simulink model "gm_UZ_EnDat_be4_segregation"  (R2023b)
settings: Solver=FixedStepAuto  StartTime=0  StopTime=0.000505  RelTol=1e-3
model workspace (MAT data in the model file):
  Select = 0
libraries: hdlsllib x74, simulink x21, hdlmdlgenlib x4, simulink_extras x1
(part 4 of 5)

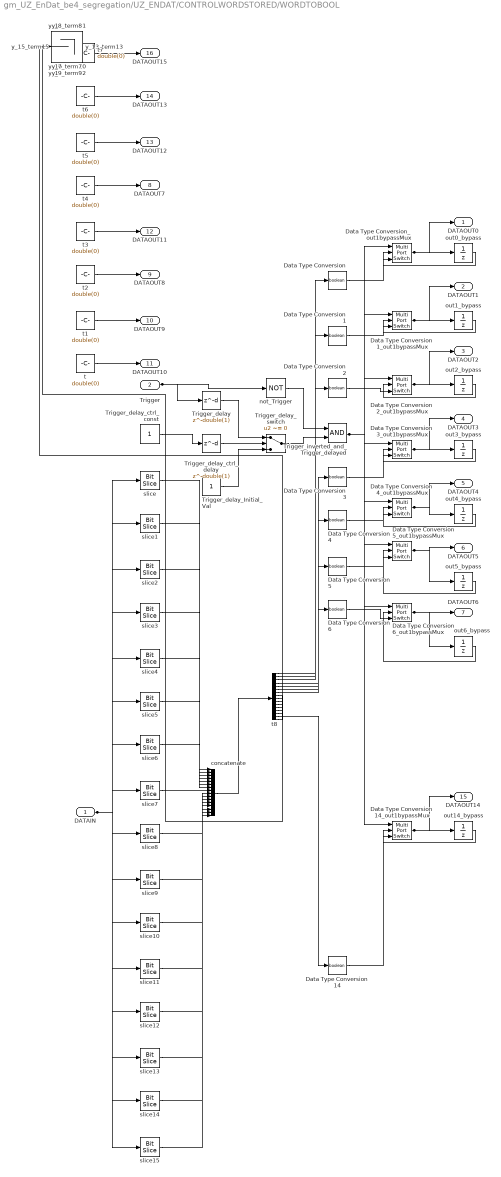
== system gm_UZ_EnDat_be4_segregation/UZ_ENDAT/CONTROLWORDSTORED/WORDTOBOOL ==
  DATAIN : Inport  OutDataTypeStr=uint16  PortDimensions=1  SampleTime=1e-08
  Trigger : Inport  Port=2  OutDataTypeStr=boolean  SampleTime=1e-08
  Data Type Conversion{,1..6,14} (8 alike) : DataTypeConversion  OutDataTypeStr=boolean  SampleTime=1e-08  SaturateOnIntegerOverflow=off  RndMeth=Floor
  Data Type Conversion14_out1bypassMux : MultiPortSwitch  DataPortOrder=Zero-based contiguous  Inputs=2  zeroidx=on  SampleTime=1e-08  SaturateOnIntegerOverflow=off  InputSameDT=off
  Data Type Conversion1_out1bypassMux : MultiPortSwitch  DataPortOrder=Zero-based contiguous  Inputs=2  zeroidx=on  SampleTime=1e-08  SaturateOnIntegerOverflow=off  InputSameDT=off
  Data Type Conversion2_out1bypassMux : MultiPortSwitch  DataPortOrder=Zero-based contiguous  Inputs=2  zeroidx=on  SampleTime=1e-08  SaturateOnIntegerOverflow=off  InputSameDT=off
  Data Type Conversion3_out1bypassMux : MultiPortSwitch  DataPortOrder=Zero-based contiguous  Inputs=2  zeroidx=on  SampleTime=1e-08  SaturateOnIntegerOverflow=off  InputSameDT=off
  Data Type Conversion4_out1bypassMux : MultiPortSwitch  DataPortOrder=Zero-based contiguous  Inputs=2  zeroidx=on  SampleTime=1e-08  SaturateOnIntegerOverflow=off  InputSameDT=off
  Data Type Conversion5_out1bypassMux : MultiPortSwitch  DataPortOrder=Zero-based contiguous  Inputs=2  zeroidx=on  SampleTime=1e-08  SaturateOnIntegerOverflow=off  InputSameDT=off
  Data Type Conversion6_out1bypassMux : MultiPortSwitch  DataPortOrder=Zero-based contiguous  Inputs=2  zeroidx=on  SampleTime=1e-08  SaturateOnIntegerOverflow=off  InputSameDT=off
  Data Type Conversion_out1bypassMux : MultiPortSwitch  DataPortOrder=Zero-based contiguous  Inputs=2  zeroidx=on  SampleTime=1e-08  SaturateOnIntegerOverflow=off  InputSameDT=off
  Trigger_delay : Delay  DelayLength=double(1)  InitialCondition=0
  Trigger_delay_Initial_Val : Constant  OutDataTypeStr=boolean  SampleTime=1e-08
  Trigger_delay_ctrl_const : Constant  OutDataTypeStr=boolean  SampleTime=1e-08
  Trigger_delay_ctrl_delay : Delay  DelayLength=double(1)  InitialCondition=0
  Trigger_delay_switch : Switch  Criteria=u2 ~= 0  Threshold=double(0)  OutDataTypeStr=boolean  SampleTime=1e-08  SaturateOnIntegerOverflow=off  InputSameDT=off
  Trigger_inverted_and_Trigger_delayed : Logic  AllPortsSameDT=off  OutDataTypeStr=boolean  SampleTime=1e-08
  concatenate : Concatenate  NumInputs=16  Mode=Multidimensional array  ConcatenateDimension=2
  not_Trigger : Logic  Operator=NOT  Inputs=1  AllPortsSameDT=off  OutDataTypeStr=boolean  SampleTime=1e-08
  out0_bypass : UnitDelay  SampleTime=1e-08
  out14_bypass : UnitDelay  SampleTime=1e-08
  out1_bypass : UnitDelay  SampleTime=1e-08
  out2_bypass : UnitDelay  SampleTime=1e-08
  out3_bypass : UnitDelay  SampleTime=1e-08
  out4_bypass : UnitDelay  SampleTime=1e-08
  out5_bypass : UnitDelay  SampleTime=1e-08
  out6_bypass : UnitDelay  SampleTime=1e-08
  slice : hdlsllib/Logic and Bit Operations/Bit Slice  lidx=double(0)  ridx=double(0)
  slice1 : hdlsllib/Logic and Bit Operations/Bit Slice  lidx=double(1)  ridx=double(1)
  slice10 : hdlsllib/Logic and Bit Operations/Bit Slice  lidx=double(10)  ridx=double(10)
  slice11 : hdlsllib/Logic and Bit Operations/Bit Slice  lidx=double(11)  ridx=double(11)
  slice12 : hdlsllib/Logic and Bit Operations/Bit Slice  lidx=double(12)  ridx=double(12)
  slice13 : hdlsllib/Logic and Bit Operations/Bit Slice  lidx=double(13)  ridx=double(13)
  slice14 : hdlsllib/Logic and Bit Operations/Bit Slice  lidx=double(14)  ridx=double(14)
  slice15 : hdlsllib/Logic and Bit Operations/Bit Slice  lidx=double(15)  ridx=double(15)
  slice2 : hdlsllib/Logic and Bit Operations/Bit Slice  lidx=double(2)  ridx=double(2)
  slice3 : hdlsllib/Logic and Bit Operations/Bit Slice  lidx=double(3)  ridx=double(3)
  slice4 : hdlsllib/Logic and Bit Operations/Bit Slice  lidx=double(4)  ridx=double(4)
  slice5 : hdlsllib/Logic and Bit Operations/Bit Slice  lidx=double(5)  ridx=double(5)
  slice6 : hdlsllib/Logic and Bit Operations/Bit Slice  lidx=double(6)  ridx=double(6)
  slice7 : hdlsllib/Logic and Bit Operations/Bit Slice  lidx=double(7)  ridx=double(7)
  slice8 : hdlsllib/Logic and Bit Operations/Bit Slice  lidx=double(8)  ridx=double(8)
  slice9 : hdlsllib/Logic and Bit Operations/Bit Slice  lidx=double(9)  ridx=double(9)
  t{,1..7} (8 alike) : Constant  Value=double(0)  OutDataTypeStr=boolean  SampleTime=1e-08
  t8 : Demux  Outputs=16
  y_10_term10 : Terminator
  y_11_term11 : Terminator
  y_12_term12 : Terminator
  y_13_term13 : Terminator
  y_15_term15 : Terminator
  y_7_term7 : Terminator
  y_8_term8 : Terminator
  y_9_term9 : Terminator
  DATAOUT0 : Outport  SampleTime=1e-08  InitialOutput=0
  DATAOUT1 : Outport  Port=2  SampleTime=1e-08  InitialOutput=0
  DATAOUT2 : Outport  Port=3  SampleTime=1e-08  InitialOutput=0
  DATAOUT3 : Outport  Port=4  SampleTime=1e-08  InitialOutput=0
  DATAOUT4 : Outport  Port=5  SampleTime=1e-08  InitialOutput=0
  DATAOUT5 : Outport  Port=6  SampleTime=1e-08  InitialOutput=0
  DATAOUT6 : Outport  Port=7  SampleTime=1e-08  InitialOutput=0
  DATAOUT7 : Outport  Port=8  SampleTime=1e-08  InitialOutput=0
  DATAOUT8 : Outport  Port=9  SampleTime=1e-08  InitialOutput=0
  DATAOUT9 : Outport  Port=10  SampleTime=1e-08  InitialOutput=0
  DATAOUT10 : Outport  Port=11  SampleTime=1e-08  InitialOutput=0
  DATAOUT11 : Outport  Port=12  SampleTime=1e-08  InitialOutput=0
  DATAOUT12 : Outport  Port=13  SampleTime=1e-08  InitialOutput=0
  DATAOUT13 : Outport  Port=14  SampleTime=1e-08  InitialOutput=0
  DATAOUT14 : Outport  Port=15  SampleTime=1e-08  InitialOutput=0
  DATAOUT15 : Outport  Port=16  SampleTime=1e-08  InitialOutput=0
  wires:
  Trigger/1 -> not_Trigger/1, Trigger_delay/1
  DATAIN/1 -> slice15/1, slice14/1, slice13/1, slice12/1, slice11/1, slice10/1, slice9/1, slice8/1, slice7/1, slice6/1, slice5/1, slice4/1, slice3/1, slice2/1, slice1/1, slice/1
  Data Type Conversion_out1bypassMux/1 -> DATAOUT0/1, out0_bypass/1
  Data Type Conversion1_out1bypassMux/1 -> DATAOUT1/1, out1_bypass/1
  Data Type Conversion2_out1bypassMux/1 -> DATAOUT2/1, out2_bypass/1
  Data Type Conversion3_out1bypassMux/1 -> DATAOUT3/1, out3_bypass/1
  Data Type Conversion4_out1bypassMux/1 -> DATAOUT4/1, out4_bypass/1
  Data Type Conversion5_out1bypassMux/1 -> DATAOUT5/1, out5_bypass/1
  Data Type Conversion6_out1bypassMux/1 -> DATAOUT6/1, out6_bypass/1
  t4/1 -> DATAOUT7/1
  t2/1 -> DATAOUT8/1
  t1/1 -> DATAOUT9/1
  t/1 -> DATAOUT10/1
  t3/1 -> DATAOUT11/1
  t5/1 -> DATAOUT12/1
  t6/1 -> DATAOUT13/1
  Data Type Conversion14_out1bypassMux/1 -> DATAOUT14/1, out14_bypass/1
  t7/1 -> DATAOUT15/1
  Trigger_delay_switch/1 -> Trigger_inverted_and_Trigger_delayed/2
  not_Trigger/1 -> Trigger_inverted_and_Trigger_delayed/1
  Trigger_inverted_and_Trigger_delayed/1 -> Data Type Conversion_out1bypassMux/1, Data Type Conversion1_out1bypassMux/1, Data Type Conversion2_out1bypassMux/1, Data Type Conversion3_out1bypassMux/1, Data Type Conversion4_out1bypassMux/1, Data Type Conversion5_out1bypassMux/1, Data Type Conversion6_out1bypassMux/1, Data Type Conversion14_out1bypassMux/1
  Trigger_delay/1 -> Trigger_delay_switch/1
  Trigger_delay_Initial_Val/1 -> Trigger_delay_switch/3
  Trigger_delay_ctrl_delay/1 -> Trigger_delay_switch/2
  concatenate/1 -> t8/1
  t8/1 -> Data Type Conversion/1
  t8/2 -> Data Type Conversion1/1
  t8/3 -> Data Type Conversion2/1
  t8/4 -> Data Type Conversion3/1
  t8/5 -> Data Type Conversion4/1
  t8/6 -> Data Type Conversion5/1
  t8/7 -> Data Type Conversion6/1
  t8/8 -> y_7_term7/1
  t8/9 -> y_8_term8/1
  t8/10 -> y_9_term9/1
  t8/11 -> y_10_term10/1
  t8/12 -> y_11_term11/1
  t8/13 -> y_12_term12/1
  t8/14 -> y_13_term13/1
  t8/15 -> Data Type Conversion14/1
  t8/16 -> y_15_term15/1
  slice/1 -> concatenate/1
  slice1/1 -> concatenate/2
  slice2/1 -> concatenate/3
  slice3/1 -> concatenate/4
  slice4/1 -> concatenate/5
  slice5/1 -> concatenate/6
  slice6/1 -> concatenate/7
  slice7/1 -> concatenate/8
  slice8/1 -> concatenate/9
  slice9/1 -> concatenate/10
  slice10/1 -> concatenate/11
  slice11/1 -> concatenate/12
  slice12/1 -> concatenate/13
  slice13/1 -> concatenate/14
  slice14/1 -> concatenate/15
  slice15/1 -> concatenate/16
  out14_bypass/1 -> Data Type Conversion14_out1bypassMux/2
  Data Type Conversion14/1 -> Data Type Conversion14_out1bypassMux/3
  out0_bypass/1 -> Data Type Conversion_out1bypassMux/2
  Data Type Conversion/1 -> Data Type Conversion_out1bypassMux/3
  out1_bypass/1 -> Data Type Conversion1_out1bypassMux/2
  Data Type Conversion1/1 -> Data Type Conversion1_out1bypassMux/3
  out2_bypass/1 -> Data Type Conversion2_out1bypassMux/2
  Data Type Conversion2/1 -> Data Type Conversion2_out1bypassMux/3
  out3_bypass/1 -> Data Type Conversion3_out1bypassMux/2
  Data Type Conversion3/1 -> Data Type Conversion3_out1bypassMux/3
  out4_bypass/1 -> Data Type Conversion4_out1bypassMux/2
  Data Type Conversion4/1 -> Data Type Conversion4_out1bypassMux/3
  out5_bypass/1 -> Data Type Conversion5_out1bypassMux/2
  Data Type Conversion5/1 -> Data Type Conversion5_out1bypassMux/3
  out6_bypass/1 -> Data Type Conversion6_out1bypassMux/2
  Data Type Conversion6/1 -> Data Type Conversion6_out1bypassMux/3
  Trigger_delay_ctrl_const/1 -> Trigger_delay_ctrl_delay/1

== system gm_UZ_EnDat_be4_segregation/UZ_ENDAT/CRC_Check/FF0 ==
  S : Inport  OutDataTypeStr=boolean  PortDimensions=1  SampleTime=1e-08
  CLK : Inport  Port=2  OutDataTypeStr=boolean  PortDimensions=1  SampleTime=1e-08
  DATA : Inport  Port=3  OutDataTypeStr=boolean  PortDimensions=1  SampleTime=1e-08
  R : Inport  Port=4  OutDataTypeStr=boolean  PortDimensions=1  SampleTime=1e-08
  Delay{,1..5} (6 alike) : Delay  DelayLength=double(1)  InitialCondition=0  SampleTime=1e-08
  Logical Operator{,1..5} (6 alike) : Logic  Operator=NAND  Inputs=3  AllPortsSameDT=off  OutDataTypeStr=boolean  SampleTime=1e-08
  Q : Outport  SampleTime=1e-08
  NQ : Outport  Port=2  SampleTime=1e-08
  wires:
  S/1 -> Logical Operator/1, Logical Operator4/1
  CLK/1 -> Logical Operator1/2, Logical Operator2/2
  R/1 -> Logical Operator3/3, Logical Operator1/3, Logical Operator5/3
  Delay1/1 -> Logical Operator/3, Logical Operator2/1, Logical Operator4/2
  Delay2/1 -> Logical Operator3/1, Logical Operator5/2
  Delay4/1 -> Q/1, Logical Operator5/1
  Delay5/1 -> NQ/1, Logical Operator4/3
  Delay3/1 -> Logical Operator/2, Logical Operator2/3
  Logical Operator2/1 -> Delay2/1
  Logical Operator3/1 -> Delay3/1
  DATA/1 -> Logical Operator3/2
  Logical Operator/1 -> Delay/1
  Logical Operator1/1 -> Delay1/1
  Delay/1 -> Logical Operator1/1
  Logical Operator5/1 -> Delay5/1
  Logical Operator4/1 -> Delay4/1

== system gm_UZ_EnDat_be4_segregation/UZ_ENDAT/CRC_Check/FF1 ==
  S : Inport  OutDataTypeStr=boolean  PortDimensions=1  SampleTime=1e-08
  CLK : Inport  Port=2  OutDataTypeStr=boolean  PortDimensions=1  SampleTime=1e-08
  DATA : Inport  Port=3  OutDataTypeStr=boolean  PortDimensions=1  SampleTime=1e-08
  R : Inport  Port=4  OutDataTypeStr=boolean  PortDimensions=1  SampleTime=1e-08
  Delay{,1..5} (6 alike) : Delay  DelayLength=double(1)  InitialCondition=0  SampleTime=1e-08
  Logical Operator{,1..5} (6 alike) : Logic  Operator=NAND  Inputs=3  AllPortsSameDT=off  OutDataTypeStr=boolean  SampleTime=1e-08
  Q : Outport  SampleTime=1e-08
  NQ : Outport  Port=2  SampleTime=1e-08
  wires:
  Logical Operator4/1 -> Delay4/1
  Logical Operator5/1 -> Delay5/1
  Delay/1 -> Logical Operator1/1
  Logical Operator1/1 -> Delay1/1
  Logical Operator/1 -> Delay/1
  DATA/1 -> Logical Operator3/2
  Logical Operator3/1 -> Delay3/1
  Logical Operator2/1 -> Delay2/1
  Delay3/1 -> Logical Operator2/3, Logical Operator/2
  Delay5/1 -> Logical Operator4/3, NQ/1
  Delay4/1 -> Logical Operator5/1, Q/1
  Delay2/1 -> Logical Operator5/2, Logical Operator3/1
  Delay1/1 -> Logical Operator4/2, Logical Operator2/1, Logical Operator/3
  R/1 -> Logical Operator5/3, Logical Operator1/3, Logical Operator3/3
  CLK/1 -> Logical Operator2/2, Logical Operator1/2
  S/1 -> Logical Operator4/1, Logical Operator/1

== system gm_UZ_EnDat_be4_segregation/UZ_ENDAT/CRC_Check/FF2 ==
  S : Inport  OutDataTypeStr=boolean  PortDimensions=1  SampleTime=1e-08
  CLK : Inport  Port=2  OutDataTypeStr=boolean  PortDimensions=1  SampleTime=1e-08
  DATA : Inport  Port=3  OutDataTypeStr=boolean  PortDimensions=1  SampleTime=1e-08
  R : Inport  Port=4  OutDataTypeStr=boolean  PortDimensions=1  SampleTime=1e-08
  Delay{,1..5} (6 alike) : Delay  DelayLength=double(1)  InitialCondition=0  SampleTime=1e-08
  Logical Operator{,1..5} (6 alike) : Logic  Operator=NAND  Inputs=3  AllPortsSameDT=off  OutDataTypeStr=boolean  SampleTime=1e-08
  Q : Outport  SampleTime=1e-08
  NQ : Outport  Port=2  SampleTime=1e-08
  wires:
  Logical Operator4/1 -> Delay4/1
  Logical Operator5/1 -> Delay5/1
  Delay/1 -> Logical Operator1/1
  Logical Operator1/1 -> Delay1/1
  Logical Operator/1 -> Delay/1
  DATA/1 -> Logical Operator3/2
  Logical Operator3/1 -> Delay3/1
  Logical Operator2/1 -> Delay2/1
  Delay3/1 -> Logical Operator2/3, Logical Operator/2
  Delay5/1 -> Logical Operator4/3, NQ/1
  Delay4/1 -> Logical Operator5/1, Q/1
  Delay2/1 -> Logical Operator5/2, Logical Operator3/1
  Delay1/1 -> Logical Operator4/2, Logical Operator2/1, Logical Operator/3
  R/1 -> Logical Operator5/3, Logical Operator1/3, Logical Operator3/3
  CLK/1 -> Logical Operator2/2, Logical Operator1/2
  S/1 -> Logical Operator4/1, Logical Operator/1

== system gm_UZ_EnDat_be4_segregation/UZ_ENDAT/CRC_Check/FF3 ==
  S : Inport  OutDataTypeStr=boolean  PortDimensions=1  SampleTime=1e-08
  CLK : Inport  Port=2  OutDataTypeStr=boolean  PortDimensions=1  SampleTime=1e-08
  DATA : Inport  Port=3  OutDataTypeStr=boolean  PortDimensions=1  SampleTime=1e-08
  R : Inport  Port=4  OutDataTypeStr=boolean  PortDimensions=1  SampleTime=1e-08
  Delay{,1..5} (6 alike) : Delay  DelayLength=double(1)  InitialCondition=0  SampleTime=1e-08
  Logical Operator{,1..5} (6 alike) : Logic  Operator=NAND  Inputs=3  AllPortsSameDT=off  OutDataTypeStr=boolean  SampleTime=1e-08
  Q : Outport  SampleTime=1e-08
  NQ : Outport  Port=2  SampleTime=1e-08
  wires:
  Logical Operator4/1 -> Delay4/1
  Logical Operator5/1 -> Delay5/1
  Delay/1 -> Logical Operator1/1
  Logical Operator1/1 -> Delay1/1
  Logical Operator/1 -> Delay/1
  DATA/1 -> Logical Operator3/2
  Logical Operator3/1 -> Delay3/1
  Logical Operator2/1 -> Delay2/1
  Delay3/1 -> Logical Operator2/3, Logical Operator/2
  Delay5/1 -> Logical Operator4/3, NQ/1
  Delay4/1 -> Logical Operator5/1, Q/1
  Delay2/1 -> Logical Operator5/2, Logical Operator3/1
  Delay1/1 -> Logical Operator4/2, Logical Operator2/1, Logical Operator/3
  R/1 -> Logical Operator5/3, Logical Operator1/3, Logical Operator3/3
  CLK/1 -> Logical Operator2/2, Logical Operator1/2
  S/1 -> Logical Operator4/1, Logical Operator/1

== system gm_UZ_EnDat_be4_segregation/UZ_ENDAT/CRC_Check/FF4 ==
  S : Inport  OutDataTypeStr=boolean  PortDimensions=1  SampleTime=1e-08
  CLK : Inport  Port=2  OutDataTypeStr=boolean  PortDimensions=1  SampleTime=1e-08
  DATA : Inport  Port=3  OutDataTypeStr=boolean  PortDimensions=1  SampleTime=1e-08
  R : Inport  Port=4  OutDataTypeStr=boolean  PortDimensions=1  SampleTime=1e-08
  Delay{,1..5} (6 alike) : Delay  DelayLength=double(1)  InitialCondition=0  SampleTime=1e-08
  Logical Operator{,1..5} (6 alike) : Logic  Operator=NAND  Inputs=3  AllPortsSameDT=off  OutDataTypeStr=boolean  SampleTime=1e-08
  Q : Outport  SampleTime=1e-08
  NQ : Outport  Port=2  SampleTime=1e-08
  wires:
  Logical Operator4/1 -> Delay4/1
  Logical Operator5/1 -> Delay5/1
  Delay/1 -> Logical Operator1/1
  Logical Operator1/1 -> Delay1/1
  Logical Operator/1 -> Delay/1
  DATA/1 -> Logical Operator3/2
  Logical Operator3/1 -> Delay3/1
  Logical Operator2/1 -> Delay2/1
  Delay3/1 -> Logical Operator2/3, Logical Operator/2
  Delay5/1 -> Logical Operator4/3, NQ/1
  Delay4/1 -> Logical Operator5/1, Q/1
  Delay2/1 -> Logical Operator5/2, Logical Operator3/1
  Delay1/1 -> Logical Operator4/2, Logical Operator2/1, Logical Operator/3
  R/1 -> Logical Operator5/3, Logical Operator1/3, Logical Operator3/3
  CLK/1 -> Logical Operator2/2, Logical Operator1/2
  S/1 -> Logical Operator4/1, Logical Operator/1

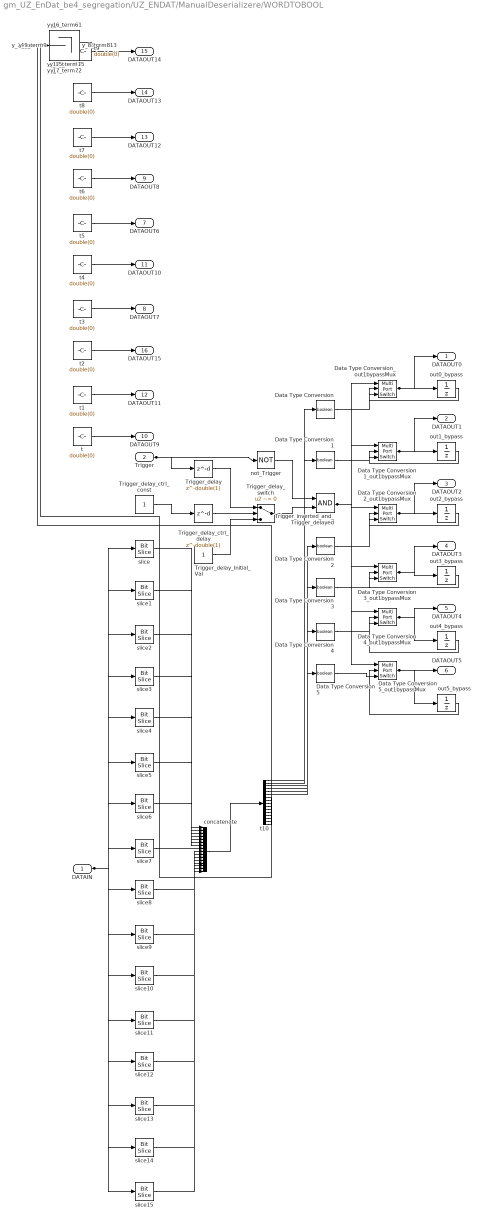
== system gm_UZ_EnDat_be4_segregation/UZ_ENDAT/ManualDeserializere/WORDTOBOOL ==
  DATAIN : Inport  OutDataTypeStr=uint16  PortDimensions=1  SampleTime=1e-08
  Trigger : Inport  Port=2  OutDataTypeStr=boolean  SampleTime=1e-08
  Data Type Conversion{,1..5} (6 alike) : DataTypeConversion  OutDataTypeStr=boolean  SampleTime=1e-08  SaturateOnIntegerOverflow=off  RndMeth=Floor
  Data Type Conversion1_out1bypassMux : MultiPortSwitch  DataPortOrder=Zero-based contiguous  Inputs=2  zeroidx=on  SampleTime=1e-08  SaturateOnIntegerOverflow=off  InputSameDT=off
  Data Type Conversion2_out1bypassMux : MultiPortSwitch  DataPortOrder=Zero-based contiguous  Inputs=2  zeroidx=on  SampleTime=1e-08  SaturateOnIntegerOverflow=off  InputSameDT=off
  Data Type Conversion3_out1bypassMux : MultiPortSwitch  DataPortOrder=Zero-based contiguous  Inputs=2  zeroidx=on  SampleTime=1e-08  SaturateOnIntegerOverflow=off  InputSameDT=off
  Data Type Conversion4_out1bypassMux : MultiPortSwitch  DataPortOrder=Zero-based contiguous  Inputs=2  zeroidx=on  SampleTime=1e-08  SaturateOnIntegerOverflow=off  InputSameDT=off
  Data Type Conversion5_out1bypassMux : MultiPortSwitch  DataPortOrder=Zero-based contiguous  Inputs=2  zeroidx=on  SampleTime=1e-08  SaturateOnIntegerOverflow=off  InputSameDT=off
  Data Type Conversion_out1bypassMux : MultiPortSwitch  DataPortOrder=Zero-based contiguous  Inputs=2  zeroidx=on  SampleTime=1e-08  SaturateOnIntegerOverflow=off  InputSameDT=off
  Trigger_delay : Delay  DelayLength=double(1)  InitialCondition=0
  Trigger_delay_Initial_Val : Constant  OutDataTypeStr=boolean  SampleTime=1e-08
  Trigger_delay_ctrl_const : Constant  OutDataTypeStr=boolean  SampleTime=1e-08
  Trigger_delay_ctrl_delay : Delay  DelayLength=double(1)  InitialCondition=0
  Trigger_delay_switch : Switch  Criteria=u2 ~= 0  Threshold=double(0)  OutDataTypeStr=boolean  SampleTime=1e-08  SaturateOnIntegerOverflow=off  InputSameDT=off
  Trigger_inverted_and_Trigger_delayed : Logic  AllPortsSameDT=off  OutDataTypeStr=boolean  SampleTime=1e-08
  concatenate : Concatenate  NumInputs=16  Mode=Multidimensional array  ConcatenateDimension=2
  not_Trigger : Logic  Operator=NOT  Inputs=1  AllPortsSameDT=off  OutDataTypeStr=boolean  SampleTime=1e-08
  out0_bypass : UnitDelay  SampleTime=1e-08
  out1_bypass : UnitDelay  SampleTime=1e-08
  out2_bypass : UnitDelay  SampleTime=1e-08
  out3_bypass : UnitDelay  SampleTime=1e-08
  out4_bypass : UnitDelay  SampleTime=1e-08
  out5_bypass : UnitDelay  SampleTime=1e-08
  slice : hdlsllib/Logic and Bit Operations/Bit Slice  lidx=double(0)  ridx=double(0)
  slice1 : hdlsllib/Logic and Bit Operations/Bit Slice  lidx=double(1)  ridx=double(1)
  slice10 : hdlsllib/Logic and Bit Operations/Bit Slice  lidx=double(10)  ridx=double(10)
  slice11 : hdlsllib/Logic and Bit Operations/Bit Slice  lidx=double(11)  ridx=double(11)
  slice12 : hdlsllib/Logic and Bit Operations/Bit Slice  lidx=double(12)  ridx=double(12)
  slice13 : hdlsllib/Logic and Bit Operations/Bit Slice  lidx=double(13)  ridx=double(13)
  slice14 : hdlsllib/Logic and Bit Operations/Bit Slice  lidx=double(14)  ridx=double(14)
  slice15 : hdlsllib/Logic and Bit Operations/Bit Slice  lidx=double(15)  ridx=double(15)
  slice2 : hdlsllib/Logic and Bit Operations/Bit Slice  lidx=double(2)  ridx=double(2)
  slice3 : hdlsllib/Logic and Bit Operations/Bit Slice  lidx=double(3)  ridx=double(3)
  slice4 : hdlsllib/Logic and Bit Operations/Bit Slice  lidx=double(4)  ridx=double(4)
  slice5 : hdlsllib/Logic and Bit Operations/Bit Slice  lidx=double(5)  ridx=double(5)
  slice6 : hdlsllib/Logic and Bit Operations/Bit Slice  lidx=double(6)  ridx=double(6)
  slice7 : hdlsllib/Logic and Bit Operations/Bit Slice  lidx=double(7)  ridx=double(7)
  slice8 : hdlsllib/Logic and Bit Operations/Bit Slice  lidx=double(8)  ridx=double(8)
  slice9 : hdlsllib/Logic and Bit Operations/Bit Slice  lidx=double(9)  ridx=double(9)
  t{,1..9} (10 alike) : Constant  Value=double(0)  OutDataTypeStr=boolean  SampleTime=1e-08
  t10 : Demux  Outputs=16
  y_10_term10 : Terminator
  y_11_term11 : Terminator
  y_12_term12 : Terminator
  y_13_term13 : Terminator
  y_14_term14 : Terminator
  y_15_term15 : Terminator
  y_6_term6 : Terminator
  y_7_term7 : Terminator
  y_8_term8 : Terminator
  y_9_term9 : Terminator
  DATAOUT0 : Outport  SampleTime=1e-08  InitialOutput=0
  DATAOUT1 : Outport  Port=2  SampleTime=1e-08  InitialOutput=0
  DATAOUT2 : Outport  Port=3  SampleTime=1e-08  InitialOutput=0
  DATAOUT3 : Outport  Port=4  SampleTime=1e-08  InitialOutput=0
  DATAOUT4 : Outport  Port=5  SampleTime=1e-08  InitialOutput=0
  DATAOUT5 : Outport  Port=6  SampleTime=1e-08  InitialOutput=0
  DATAOUT6 : Outport  Port=7  SampleTime=1e-08  InitialOutput=0
  DATAOUT7 : Outport  Port=8  SampleTime=1e-08  InitialOutput=0
  DATAOUT8 : Outport  Port=9  SampleTime=1e-08  InitialOutput=0
  DATAOUT9 : Outport  Port=10  SampleTime=1e-08  InitialOutput=0
  DATAOUT10 : Outport  Port=11  SampleTime=1e-08  InitialOutput=0
  DATAOUT11 : Outport  Port=12  SampleTime=1e-08  InitialOutput=0
  DATAOUT12 : Outport  Port=13  SampleTime=1e-08  InitialOutput=0
  DATAOUT13 : Outport  Port=14  SampleTime=1e-08  InitialOutput=0
  DATAOUT14 : Outport  Port=15  SampleTime=1e-08  InitialOutput=0
  DATAOUT15 : Outport  Port=16  SampleTime=1e-08  InitialOutput=0
  wires:
  Trigger/1 -> not_Trigger/1, Trigger_delay/1
  DATAIN/1 -> slice15/1, slice14/1, slice13/1, slice12/1, slice11/1, slice10/1, slice9/1, slice8/1, slice7/1, slice6/1, slice5/1, slice4/1, slice3/1, slice2/1, slice1/1, slice/1
  Data Type Conversion_out1bypassMux/1 -> DATAOUT0/1, out0_bypass/1
  Data Type Conversion1_out1bypassMux/1 -> DATAOUT1/1, out1_bypass/1
  Data Type Conversion2_out1bypassMux/1 -> DATAOUT2/1, out2_bypass/1
  Data Type Conversion3_out1bypassMux/1 -> DATAOUT3/1, out3_bypass/1
  Data Type Conversion4_out1bypassMux/1 -> DATAOUT4/1, out4_bypass/1
  Data Type Conversion5_out1bypassMux/1 -> DATAOUT5/1, out5_bypass/1
  t5/1 -> DATAOUT6/1
  t3/1 -> DATAOUT7/1
  t6/1 -> DATAOUT8/1
  t/1 -> DATAOUT9/1
  t4/1 -> DATAOUT10/1
  t1/1 -> DATAOUT11/1
  t7/1 -> DATAOUT12/1
  t8/1 -> DATAOUT13/1
  t9/1 -> DATAOUT14/1
  t2/1 -> DATAOUT15/1
  Trigger_delay_switch/1 -> Trigger_inverted_and_Trigger_delayed/2
  not_Trigger/1 -> Trigger_inverted_and_Trigger_delayed/1
  Trigger_inverted_and_Trigger_delayed/1 -> Data Type Conversion_out1bypassMux/1, Data Type Conversion1_out1bypassMux/1, Data Type Conversion2_out1bypassMux/1, Data Type Conversion3_out1bypassMux/1, Data Type Conversion4_out1bypassMux/1, Data Type Conversion5_out1bypassMux/1
  Trigger_delay/1 -> Trigger_delay_switch/1
  Trigger_delay_Initial_Val/1 -> Trigger_delay_switch/3
  Trigger_delay_ctrl_const/1 -> Trigger_delay_ctrl_delay/1
  Trigger_delay_ctrl_delay/1 -> Trigger_delay_switch/2
  concatenate/1 -> t10/1
  t10/1 -> Data Type Conversion/1
  t10/2 -> Data Type Conversion1/1
  t10/3 -> Data Type Conversion2/1
  t10/4 -> Data Type Conversion3/1
  t10/5 -> Data Type Conversion4/1
  t10/6 -> Data Type Conversion5/1
  t10/7 -> y_6_term6/1
  t10/8 -> y_7_term7/1
  t10/9 -> y_8_term8/1
  t10/10 -> y_9_term9/1
  t10/11 -> y_10_term10/1
  t10/12 -> y_11_term11/1
  t10/13 -> y_12_term12/1
  t10/14 -> y_13_term13/1
  t10/15 -> y_14_term14/1
  t10/16 -> y_15_term15/1
  slice/1 -> concatenate/1
  slice1/1 -> concatenate/2
  slice2/1 -> concatenate/3
  slice3/1 -> concatenate/4
  slice4/1 -> concatenate/5
  slice5/1 -> concatenate/6
  slice6/1 -> concatenate/7
  slice7/1 -> concatenate/8
  slice8/1 -> concatenate/9
  slice9/1 -> concatenate/10
  slice10/1 -> concatenate/11
  slice11/1 -> concatenate/12
  slice12/1 -> concatenate/13
  slice13/1 -> concatenate/14
  slice14/1 -> concatenate/15
  slice15/1 -> concatenate/16
  out0_bypass/1 -> Data Type Conversion_out1bypassMux/2
  Data Type Conversion/1 -> Data Type Conversion_out1bypassMux/3
  out1_bypass/1 -> Data Type Conversion1_out1bypassMux/2
  Data Type Conversion1/1 -> Data Type Conversion1_out1bypassMux/3
  out2_bypass/1 -> Data Type Conversion2_out1bypassMux/2
  Data Type Conversion2/1 -> Data Type Conversion2_out1bypassMux/3
  out3_bypass/1 -> Data Type Conversion3_out1bypassMux/2
  Data Type Conversion3/1 -> Data Type Conversion3_out1bypassMux/3
  out4_bypass/1 -> Data Type Conversion4_out1bypassMux/2
  Data Type Conversion4/1 -> Data Type Conversion4_out1bypassMux/3
  out5_bypass/1 -> Data Type Conversion5_out1bypassMux/2
  Data Type Conversion5/1 -> Data Type Conversion5_out1bypassMux/3

== system gm_UZ_EnDat_be4_segregation/UZ_ENDAT/ManualDeserializere/ramwatcher ==
  In1 : Inport  OutMin=0  OutMax=32000  OutDataTypeStr=uint16  PortDimensions=1  SampleTime=1e-08  LockScale=on
  In2 : Inport  Port=2  OutMin=0  OutMax=1  OutDataTypeStr=fixdt(0, 1, 0)  PortDimensions=1  SampleTime=1e-08  LockScale=on
  Trigger : Inport  Port=3  OutDataTypeStr=boolean  SampleTime=1e-08
  Increment Stored Integer : Subsystem  mask(Stored Integer Value Increment){}
      mask help: Simulink:masks:StoredIntegerValueIncrement_MD
      mask Display: disp('Q++')
  Product : Product  Inputs=**  OutDataTypeStr=uint16  SampleTime=1e-08
  Product_out1bypassMux : MultiPortSwitch  DataPortOrder=Zero-based contiguous  Inputs=2  zeroidx=on  OutDataTypeStr=uint16  SampleTime=1e-08  SaturateOnIntegerOverflow=off  InputSameDT=off
  Trigger_delay : Delay  DelayLength=double(1)  InitialCondition=0
  Trigger_delayed_inverted_and_Trigger : Logic  AllPortsSameDT=off  OutDataTypeStr=boolean  SampleTime=1e-08
  not_Trigger_delayed : Logic  Operator=NOT  Inputs=1  AllPortsSameDT=off  OutDataTypeStr=boolean  SampleTime=1e-08
  out0_bypass : UnitDelay  InitialCondition="fi(0,0,16,0,\"hex\",\"0000\")"  SampleTime=1e-08
  SEL : Outport  SampleTime=1e-08  InitialOutput=0
  wires:
  Trigger/1 -> Trigger_delayed_inverted_and_Trigger/2, Trigger_delay/1
  In1/1 -> Increment Stored Integer/1(u)
  In2/1 -> Product/2
  Product_out1bypassMux/1 -> SEL/1, out0_bypass/1
  Trigger_delay/1 -> not_Trigger_delayed/1
  not_Trigger_delayed/1 -> Trigger_delayed_inverted_and_Trigger/1
  Increment Stored Integer/1(y) -> Product/1
  Trigger_delayed_inverted_and_Trigger/1 -> Product_out1bypassMux/1
  out0_bypass/1 -> Product_out1bypassMux/2
  Product/1 -> Product_out1bypassMux/3

== system gm_UZ_EnDat_be4_segregation/UZ_ENDAT/ManualSerialize/CLKCNTER_RECIEVE ==
  CLK : Inport  OutDataTypeStr=boolean  PortDimensions=1  SampleTime=1e-08
  CLK2CNT : Inport  Port=2  OutDataTypeStr=boolean  PortDimensions=1  SampleTime=1e-08
  ResetCNT : Inport  Port=3  OutDataTypeStr=boolean  PortDimensions=1  SampleTime=1e-08
  Delay1 : Delay  DelayLength=double(1)  InitialCondition=0  SampleTime=1e-08
  Delay1_enbsw : Switch  Criteria=u2 ~= 0  Threshold=double(0)  OutDataTypeStr=uint32  SampleTime=1e-08  SaturateOnIntegerOverflow=off  InputSameDT=off
  Positional_Counter : Subsystem
  SetZero32 : Subsystem
  delayMatch : Delay  DelayLength=double(2)  InitialCondition=0  SampleTime=1e-08
  delayMatch1 : Delay  DelayLength=double(2)  InitialCondition=0  SampleTime=1e-08
  stateControl : Constant  OutDataTypeStr=boolean  SampleTime=1e-08
  CNT : Outport  SampleTime=1e-08
  wires:
  CLK/1 -> delayMatch/1
  stateControl/1 -> delayMatch1/1
  ResetCNT/1 -> SetZero32/2(setzero)
  delayMatch/1 -> SetZero32/3(Trigger)
  Positional_Counter/1(divider) -> SetZero32/1(valin)
  delayMatch1/1 -> Delay1_enbsw/2
  CLK2CNT/1 -> Positional_Counter/2(Trigger)
  Delay1/1 -> Delay1_enbsw/3, Positional_Counter/1(valueout), CNT/1
  SetZero32/1(valueout) -> Delay1_enbsw/1
  Delay1_enbsw/1 -> Delay1/1

== system gm_UZ_EnDat_be4_segregation/UZ_ENDAT/ManualSerialize/SetZero64 ==
  valin : Inport  OutDataTypeStr=fixdt(0, 64, 0)  PortDimensions=1  SampleTime=1e-08
  setzero : Inport  Port=2  OutDataTypeStr=boolean  PortDimensions=1  SampleTime=1e-08
  Trigger : Inport  Port=3  OutDataTypeStr=boolean  SampleTime=1e-08
  Constant1 : Constant  OutDataTypeStr=fixdt(0, 1, 0)  SampleTime=1e-08
  Constant2 : Constant  Value=0  OutDataTypeStr=fixdt(0, 1, 0)  SampleTime=1e-08
  Index Vector1 : MultiPortSwitch  DataPortOrder=Zero-based contiguous  Inputs=2  DiagnosticForDefault=None  zeroidx=on  OutDataTypeStr=fixdt(0, 1, 0)  SampleTime=1e-08  SaturateOnIntegerOverflow=off  InputSameDT=off
  Product : Product  Inputs=**  OutDataTypeStr=fixdt(0, 64, 0)  SaturateOnIntegerOverflow=on  SampleTime=1e-08
  Product_out1bypassMux : MultiPortSwitch  DataPortOrder=Zero-based contiguous  Inputs=2  zeroidx=on  OutDataTypeStr=fixdt(0, 64, 0)  SampleTime=1e-08  SaturateOnIntegerOverflow=off  InputSameDT=off
  Trigger_delay : Delay  DelayLength=double(1)  InitialCondition=0
  Trigger_delay_Initial_Val : Constant  OutDataTypeStr=boolean  SampleTime=1e-08
  Trigger_delay_ctrl_const : Constant  OutDataTypeStr=boolean  SampleTime=1e-08
  Trigger_delay_ctrl_delay : Delay  DelayLength=double(1)  InitialCondition=0
  Trigger_delay_switch : Switch  Criteria=u2 ~= 0  Threshold=double(0)  OutDataTypeStr=boolean  SampleTime=1e-08  SaturateOnIntegerOverflow=off  InputSameDT=off
  Trigger_delayed_inverted_and_Trigger : Logic  AllPortsSameDT=off  OutDataTypeStr=boolean  SampleTime=1e-08
  delayMatch{,1..5} (6 alike) : Delay  DelayLength=double(2)  InitialCondition=0
  not_Trigger_delayed : Logic  Operator=NOT  Inputs=1  AllPortsSameDT=off  OutDataTypeStr=boolean  SampleTime=1e-08
  out0_bypass : UnitDelay  InitialCondition=double(0)  SampleTime=1e-08
  out0_bypass_Initial_Val : Constant  Value="fi(0,0,64,0,\"hex\",\"0000000000000001\")"  OutDataTypeStr=fixdt(0, 64, 0)  SampleTime=1e-08
  out0_bypass_ctrl_const : Constant  OutDataTypeStr=boolean  SampleTime=1e-08
  out0_bypass_ctrl_delay : Delay  DelayLength=double(1)  InitialCondition=0
  out0_bypass_switch : Switch  Criteria=u2 ~= 0  Threshold=double(0)  OutDataTypeStr=fixdt(0, 64, 0)  SampleTime=1e-08  SaturateOnIntegerOverflow=off  InputSameDT=off
  valueout : Outport  SampleTime=1e-08  InitialOutput=0  VectorParamsAs1DForOutWhenUnconnected=off
  wires:
  Trigger/1 -> Trigger_delayed_inverted_and_Trigger/2, Trigger_delay/1
  valin/1 -> Product/2
  setzero/1 -> Index Vector1/1
  Trigger_delay_switch/1 -> not_Trigger_delayed/1
  not_Trigger_delayed/1 -> Trigger_delayed_inverted_and_Trigger/1
  Trigger_delay/1 -> Trigger_delay_switch/1
  delayMatch1/1 -> Trigger_delay_switch/3
  delayMatch/1 -> Trigger_delay_switch/2
  Index Vector1/1 -> Product/1
  delayMatch2/1 -> Index Vector1/2
  delayMatch3/1 -> Index Vector1/3
  Trigger_delay_ctrl_delay/1 -> delayMatch/1
  Trigger_delay_Initial_Val/1 -> delayMatch1/1
  Constant1/1 -> delayMatch2/1
  Constant2/1 -> delayMatch3/1
  out0_bypass_ctrl_delay/1 -> delayMatch4/1
  out0_bypass_Initial_Val/1 -> delayMatch5/1
  Product_out1bypassMux/1 -> out0_bypass/1, valueout/1
  out0_bypass/1 -> out0_bypass_switch/1
  delayMatch4/1 -> out0_bypass_switch/2
  delayMatch5/1 -> out0_bypass_switch/3
  Trigger_delayed_inverted_and_Trigger/1 -> Product_out1bypassMux/1
  Product/1 -> Product_out1bypassMux/3
  out0_bypass_switch/1 -> Product_out1bypassMux/2
  out0_bypass_ctrl_const/1 -> out0_bypass_ctrl_delay/1
  Trigger_delay_ctrl_const/1 -> Trigger_delay_ctrl_delay/1

== system gm_UZ_EnDat_be4_segregation/UZ_ENDAT/ManualSerialize/Storage16 ==
  Data : Inport  OutDataTypeStr=fixdt(0, 64, 0)  PortDimensions=1  SampleTime=1e-08
  Write : Inport  Port=2  OutDataTypeStr=boolean  PortDimensions=1  SampleTime=1e-08
  Compare To Zero : Subsystem  mask(Compare To Zero){relop===, OutDataTypeStr=boolean, ZeroCross=on}
      mask prompts: relop "Simulink:masks:Operator_MP"; OutDataTypeStr "Simulink:masks:OutputDataType_MP"; ZeroCross "Simulink:masks:EnableZerocrossingDetection_MP"
      mask help: Simulink:masks:CompareToZero_MD
      mask init:
      | OutDataTypeStr = 'boolean';
      | ZeroCross = 'on';
      | blkName = 'UZ_EnDat_be4_segregation/UZ_ENDAT/ManualSerialize/Storage16/Compare\nTo Zero';
      | relop = '==';
      | setValue = 'boolean';
      mask TypeOptions relop: == | ~= | < | <= | >= | >
      mask TypeOptions OutDataTypeStr: Simulink:masks:uint8 | Simulink:masks:boolean
      mask Callback ZeroCross: sl('zeroCrossEnable', gcbh);
      mask Display: disp([relop,' 0'])
  Logical Operator : Logic  Operator=NOT  Inputs=1  AllPortsSameDT=off  OutDataTypeStr=boolean  SampleTime=1e-08
  Logical Operator1 : Logic  Inputs=3  AllPortsSameDT=off  OutDataTypeStr=boolean  SampleTime=1e-08
  Logical Operator2 : Logic  Operator=NOT  Inputs=1  AllPortsSameDT=off  OutDataTypeStr=boolean  SampleTime=1e-08
  Logical Operator3 : Logic  AllPortsSameDT=off  OutDataTypeStr=boolean  SampleTime=1e-08
  Relational Operator : RelationalOperator  Operator===  OutDataTypeStr=boolean  SampleTime=1e-08  InputSameDT=off
  Single Port RAM System : hdlsllib/HDL RAMs/Single Port RAM System  RAMType=Single port  AsyncRead=off  WriteOutputValue=Old data  RAMInitialValue=0  allowBusInputs=off  WritesHaveOutput=on  NumReads=0  NumWrites=1  SimulateUsing=Code generation
  adress : Constant  Value=6  OutDataTypeStr=uint8  SampleTime=1e-08
  out : Outport  SampleTime=1e-08
  wrok : Outport  Port=2  OutDataTypeStr=boolean  SampleTime=1e-08
  wires:
  Data/1 -> Compare To Zero/1(u), Relational Operator/2, Single Port RAM System/1
  Write/1 -> Logical Operator1/1
  Compare To Zero/1(y) -> Logical Operator2/1
  Logical Operator2/1 -> Logical Operator3/2, Logical Operator1/3
  Logical Operator3/1 -> wrok/1
  adress/1 -> Single Port RAM System/2
  Relational Operator/1 -> Logical Operator/1, Logical Operator3/1
  Single Port RAM System/1 -> Relational Operator/1, out/1
  Logical Operator/1 -> Logical Operator1/2
  Logical Operator1/1 -> Single Port RAM System/3

== system gm_UZ_EnDat_be4_segregation/UZ_ENDAT/ManualSerialize/Triggered Subsystem ==
  In1 : Inport  OutDataTypeStr=boolean  PortDimensions=1  SampleTime=1e-08
  valueout : Inport  Port=2  OutDataTypeStr=fixdt(0, 64, 0)  PortDimensions=1  SampleTime=1e-08
  Trigger : Inport  Port=3  OutDataTypeStr=boolean  SampleTime=1e-08
  Bit Clear : simulink/Logic and Bit Operations/Bit Clear  iBit=double(48)
  Bit Set : simulink/Logic and Bit Operations/Bit Set  iBit=double(48)
  Bit Shift : hdlsllib/Logic and Bit Operations/Bit Shift  mode=Shift Right Logical  N=double(1)
  Bit Shift_out1bypassMux : MultiPortSwitch  DataPortOrder=Zero-based contiguous  Inputs=2  zeroidx=on  OutDataTypeStr=fixdt(0, 64, 0)  SampleTime=1e-08  SaturateOnIntegerOverflow=off  InputSameDT=off
  Switch : Switch  Criteria=u2 ~= 0  Threshold=double(0)  OutDataTypeStr=fixdt(0, 64, 0)  SampleTime=1e-08  SaturateOnIntegerOverflow=off  InputSameDT=off
  Trigger_delay : Delay  DelayLength=double(1)  InitialCondition=0
  Trigger_delay_Initial_Val : Constant  OutDataTypeStr=boolean  SampleTime=1e-08
  Trigger_delay_ctrl_const : Constant  OutDataTypeStr=boolean  SampleTime=1e-08
  Trigger_delay_ctrl_delay : Delay  DelayLength=double(1)  InitialCondition=0
  Trigger_delay_switch : Switch  Criteria=u2 ~= 0  Threshold=double(0)  OutDataTypeStr=boolean  SampleTime=1e-08  SaturateOnIntegerOverflow=off  InputSameDT=off
  Trigger_delayed_inverted_and_Trigger : Logic  AllPortsSameDT=off  OutDataTypeStr=boolean  SampleTime=1e-08
  delayMatch : Delay  DelayLength=double(2)  InitialCondition=0
  delayMatch1 : Delay  DelayLength=double(2)  InitialCondition=0
  not_Trigger_delayed : Logic  Operator=NOT  Inputs=1  AllPortsSameDT=off  OutDataTypeStr=boolean  SampleTime=1e-08
  out0_bypass : UnitDelay  InitialCondition="fi(0,0,64,0,\"hex\",\"0000000000000000\")"  SampleTime=1e-08
  valin : Outport  SampleTime=1e-08  InitialOutput=0
  wires:
  Trigger/1 -> Trigger_delayed_inverted_and_Trigger/2, Trigger_delay/1
  In1/1 -> Switch/2
  valueout/1 -> Bit Set/1, Bit Clear/1
  Trigger_delay_switch/1 -> not_Trigger_delayed/1
  not_Trigger_delayed/1 -> Trigger_delayed_inverted_and_Trigger/1
  Trigger_delay/1 -> Trigger_delay_switch/1
  delayMatch1/1 -> Trigger_delay_switch/3
  delayMatch/1 -> Trigger_delay_switch/2
  Bit Clear/1 -> Switch/3
  Bit Set/1 -> Switch/1
  Switch/1 -> Bit Shift/1
  Trigger_delay_ctrl_delay/1 -> delayMatch/1
  Trigger_delay_Initial_Val/1 -> delayMatch1/1
  Bit Shift_out1bypassMux/1 -> out0_bypass/1, valin/1
  Trigger_delayed_inverted_and_Trigger/1 -> Bit Shift_out1bypassMux/1
  out0_bypass/1 -> Bit Shift_out1bypassMux/2
  Bit Shift/1 -> Bit Shift_out1bypassMux/3
  Trigger_delay_ctrl_const/1 -> Trigger_delay_ctrl_delay/1

== system gm_UZ_EnDat_be4_segregation/UZ_ENDAT/Storage16/Compare To Zero ==
  u : Inport  OutDataTypeStr=fixdt(0,16,0,'DataTypeOverride', 'Off')  SampleTime=1e-08
  Compare : RelationalOperator  Operator===  OutDataTypeStr=boolean
  Constant : Constant  DisableCoverage=on  Value=0  OutDataTypeStr=Inherit: Inherit via back propagation  SampleTime=-1  PreserveConstantTs=on
  y : Outport  SampleTime=1e-08
  wires:
  u/1 -> Compare/1
  Compare/1 -> y/1
  Constant/1 -> Compare/2

== system gm_UZ_EnDat_be4_segregation/UZ_ENDAT/Subsystem/CLKCNTERBOOTUP ==
  CLK : Inport  OutDataTypeStr=boolean  PortDimensions=1  SampleTime=1e-08
  CLK2CNT : Inport  Port=2  OutDataTypeStr=boolean  PortDimensions=1  SampleTime=1e-08
  ResetCNT : Inport  Port=3  OutDataTypeStr=boolean  PortDimensions=1  SampleTime=1e-08
  Delay1 : Delay  DelayLength=double(1)  InitialCondition=0  SampleTime=1e-08
  Positional_Counter : Subsystem
  SetZero64 : Subsystem
  CNT : Outport  SampleTime=1e-08
  wires:
  Delay1/1 -> CNT/1, Positional_Counter/1(valueout)
  SetZero64/1(valueout) -> Delay1/1
  CLK2CNT/1 -> Positional_Counter/2(Trigger)
  ResetCNT/1 -> SetZero64/2(setzero)
  CLK/1 -> SetZero64/3(Trigger)
  Positional_Counter/1(divider) -> SetZero64/1(valin)

== system gm_UZ_EnDat_be4_segregation/UZ_ENDAT/Subsystem/ManualDeserializere ==
  CLK : Inport  OutDataTypeStr=boolean  PortDimensions=1  SampleTime=1e-08
  SLOWCLCK : Inport  Port=2  OutDataTypeStr=boolean  PortDimensions=1  SampleTime=1e-08
  DATA : Inport  Port=3  OutDataTypeStr=uint16  PortDimensions=1  SampleTime=1e-08
  reset : Inport  Port=4  OutDataTypeStr=boolean  PortDimensions=1  SampleTime=1e-08
  14 : Inport  Port=5  OutDataTypeStr=boolean  PortDimensions=1  SampleTime=1e-08
  Constant3 : Constant  Value=0  OutDataTypeStr=boolean  SampleTime=1e-08
  Data Type Conversion : DataTypeConversion  OutDataTypeStr=fixdt(0, 1, 0)  SampleTime=1e-08  SaturateOnIntegerOverflow=off  RndMeth=Floor
  Delay : Delay  DelayLength=double(1)  InitialCondition=0  SampleTime=1e-08
  Delay1 : Delay  DelayLength=double(1)  InitialCondition=0  SampleTime=1e-08
  Logical Operator : Logic  Operator=NOT  Inputs=1  AllPortsSameDT=off  OutDataTypeStr=boolean  SampleTime=1e-08
  Multiport Switch : MultiPortSwitch  Inputs=16  DataPortForDefault=Additional data port  DiagnosticForDefault=None  SampleTime=1e-08  SaturateOnIntegerOverflow=off  InputSameDT=off
  Switch : Switch  Criteria=u2 ~= 0  Threshold=double(0)  OutDataTypeStr=boolean  SampleTime=1e-08  SaturateOnIntegerOverflow=off  InputSameDT=off
  WORDTOBOOL : Subsystem
  ramwatcher : Subsystem
  valin : Outport  SampleTime=1e-08
  wires:
  CLK/1 -> WORDTOBOOL/2(Trigger)
  SLOWCLCK/1 -> Switch/1, Delay/1
  DATA/1 -> WORDTOBOOL/1(DATAIN)
  reset/1 -> Logical Operator/1
  14/1 -> Switch/2
  Constant3/1 -> Multiport Switch/18
  Delay/1 -> Switch/3
  Logical Operator/1 -> Data Type Conversion/1
  Multiport Switch/1 -> valin/1
  WORDTOBOOL/1(DATAOUT0) -> Multiport Switch/17
  WORDTOBOOL/2(DATAOUT1) -> Multiport Switch/16
  WORDTOBOOL/3(DATAOUT2) -> Multiport Switch/15
  WORDTOBOOL/4(DATAOUT3) -> Multiport Switch/14
  WORDTOBOOL/5(DATAOUT4) -> Multiport Switch/13
  WORDTOBOOL/6(DATAOUT5) -> Multiport Switch/12
  WORDTOBOOL/7(DATAOUT6) -> Multiport Switch/11
  WORDTOBOOL/8(DATAOUT7) -> Multiport Switch/10
  WORDTOBOOL/9(DATAOUT8) -> Multiport Switch/9
  WORDTOBOOL/10(DATAOUT9) -> Multiport Switch/8
  WORDTOBOOL/11(DATAOUT10) -> Multiport Switch/7
  WORDTOBOOL/12(DATAOUT11) -> Multiport Switch/6
  WORDTOBOOL/13(DATAOUT12) -> Multiport Switch/5
  WORDTOBOOL/14(DATAOUT13) -> Multiport Switch/4
  WORDTOBOOL/15(DATAOUT14) -> Multiport Switch/3
  WORDTOBOOL/16(DATAOUT15) -> Multiport Switch/2
  ramwatcher/1(SEL) -> Multiport Switch/1, Delay1/1
  Data Type Conversion/1 -> ramwatcher/2(In2)
  Switch/1 -> ramwatcher/3(Trigger)
  Delay1/1 -> ramwatcher/1(In1)

== system gm_UZ_EnDat_be4_segregation/UZ_ENDAT/Subsystem/OUTPUTCONTROLCONTINIOUS ==
  CLKCNT : Inport  OutDataTypeStr=fixdt(0, 64, 0)  PortDimensions=1  SampleTime=1e-08
  CLKS2DATAFLOWCHG : Inport  Port=2  OutDataTypeStr=uint32  PortDimensions=1  SampleTime=1e-08
  CLK2ENDOFTRANSMISSION : Inport  Port=3  OutDataTypeStr=uint32  PortDimensions=1  SampleTime=1e-08
  OPENCOM : Inport  Port=4  OutDataTypeStr=boolean  PortDimensions=1  SampleTime=1e-08
  Logical Operator : Logic  Operator=OR  AllPortsSameDT=off  OutDataTypeStr=boolean  SampleTime=1e-08
  Logical Operator6 : Logic  Operator=NOT  Inputs=1  AllPortsSameDT=off  OutDataTypeStr=boolean  SampleTime=1e-08
  Relational Operator : RelationalOperator  Operator=<=  OutDataTypeStr=boolean  SampleTime=1e-08  InputSameDT=off
  Relational Operator1 : RelationalOperator  OutDataTypeStr=boolean  SampleTime=1e-08  InputSameDT=off
  CLKOFF : Outport  OutDataTypeStr=boolean  SampleTime=1e-08
  DATAINV : Outport  Port=2  OutDataTypeStr=boolean  SampleTime=1e-08
  RESETCNT : Outport  Port=3  OutDataTypeStr=boolean  SampleTime=1e-08
  wires:
  CLKCNT/1 -> Relational Operator1/1, Relational Operator/1
  CLKS2DATAFLOWCHG/1 -> Relational Operator/2
  CLK2ENDOFTRANSMISSION/1 -> Relational Operator1/2
  OPENCOM/1 -> Logical Operator6/1
  Logical Operator/1 -> CLKOFF/1
  Logical Operator6/1 -> Logical Operator/1
  Relational Operator/1 -> DATAINV/1
  Relational Operator1/1 -> Logical Operator/2, RESETCNT/1

== system gm_UZ_EnDat_be4_segregation/UZ_ENDAT/ramselektor/Delay ==
  in0 : Inport  OutDataTypeStr=fixdt(0,4,0,'DataTypeOverride', 'Off')  SampleTime=1e-08
  Trigger_emulated : EnablePort  OutDataTypeStr=boolean
  Delay : Delay  DelayLength=double(99)  InitialCondition=0
  out0 : Outport  OutDataTypeStr=fixdt(0,4,0,'DataTypeOverride', 'Off')  SampleTime=1e-08  InitialOutput=0
  wires:
  Delay/1 -> out0/1
  in0/1 -> Delay/1

== system gm_UZ_EnDat_be4_segregation/UZ_ENDAT/ramselektor/Increment Stored Integer ==
  u : Inport  OutDataTypeStr=fixdt(0,4,0,'DataTypeOverride', 'Off')  SampleTime=1e-08
  FixPt Constant : Constant  DisableCoverage=on  OutDataTypeStr=Inherit: Inherit via back propagation  SampleTime=-1
  FixPt Data Type Duplicate : DataTypeDuplicate  DisableCoverage=on  NumInputPorts=3
  FixPt Gateway In : DataTypeConversion  DisableCoverage=on  ConvertRealWorld=Stored Integer (SI)  SaturateOnIntegerOverflow=off  RndMeth=Floor
  FixPt Sum1 : Sum  OutDataTypeStr=Inherit: Inherit via back propagation  InputSameDT=on  LockScale=on
  sigspec : SignalSpecification  OutDataTypeStr=fixdt(0, 4, 0)  Dimensions=1
  y : Outport  SampleTime=1e-08  InitialOutput=0
  wires:
  u/1 -> FixPt Sum1/1, FixPt Data Type Duplicate/2
  FixPt Constant/1 -> sigspec/1
  FixPt Gateway In/1 -> FixPt Sum1/2, FixPt Data Type Duplicate/3
  FixPt Sum1/1 -> FixPt Data Type Duplicate/1, y/1
  sigspec/1 -> FixPt Gateway In/1

== system gm_UZ_EnDat_be4_segregation/UZ_ENDAT/5timestorage/Storage20/Compare To Zero ==
  u : Inport  OutDataTypeStr=fixdt(0,64,0,'DataTypeOverride', 'Off')  SampleTime=1e-08
  Compare : RelationalOperator  Operator===  OutDataTypeStr=boolean
  Constant : Constant  DisableCoverage=on  Value=0  OutDataTypeStr=Inherit: Inherit via back propagation  SampleTime=-1  PreserveConstantTs=on
  y : Outport  SampleTime=1e-08
  wires:
  u/1 -> Compare/1
  Compare/1 -> y/1
  Constant/1 -> Compare/2

== system gm_UZ_EnDat_be4_segregation/UZ_ENDAT/5timestorage/Storage21/Compare To Zero ==
  u : Inport  OutDataTypeStr=fixdt(0,64,0,'DataTypeOverride', 'Off')  SampleTime=1e-08
  Compare : RelationalOperator  Operator===  OutDataTypeStr=boolean
  Constant : Constant  DisableCoverage=on  Value=0  OutDataTypeStr=Inherit: Inherit via back propagation  SampleTime=-1  PreserveConstantTs=on
  y : Outport  SampleTime=1e-08
  wires:
  u/1 -> Compare/1
  Compare/1 -> y/1
  Constant/1 -> Compare/2

== system gm_UZ_EnDat_be4_segregation/UZ_ENDAT/5timestorage/Storage22/Compare To Zero ==
  u : Inport  OutDataTypeStr=fixdt(0,64,0,'DataTypeOverride', 'Off')  SampleTime=1e-08
  Compare : RelationalOperator  Operator===  OutDataTypeStr=boolean
  Constant : Constant  DisableCoverage=on  Value=0  OutDataTypeStr=Inherit: Inherit via back propagation  SampleTime=-1  PreserveConstantTs=on
  y : Outport  SampleTime=1e-08
  wires:
  u/1 -> Compare/1
  Compare/1 -> y/1
  Constant/1 -> Compare/2

== system gm_UZ_EnDat_be4_segregation/UZ_ENDAT/5timestorage/Storage23/Compare To Zero ==
  u : Inport  OutDataTypeStr=fixdt(0,64,0,'DataTypeOverride', 'Off')  SampleTime=1e-08
  Compare : RelationalOperator  Operator===  OutDataTypeStr=boolean
  Constant : Constant  DisableCoverage=on  Value=0  OutDataTypeStr=Inherit: Inherit via back propagation  SampleTime=-1  PreserveConstantTs=on
  y : Outport  SampleTime=1e-08
  wires:
  u/1 -> Compare/1
  Compare/1 -> y/1
  Constant/1 -> Compare/2

== system gm_UZ_EnDat_be4_segregation/UZ_ENDAT/5timestorage/Storage24/Compare To Zero ==
  u : Inport  OutDataTypeStr=fixdt(0,64,0,'DataTypeOverride', 'Off')  SampleTime=1e-08
  Compare : RelationalOperator  Operator===  OutDataTypeStr=boolean
  Constant : Constant  DisableCoverage=on  Value=0  OutDataTypeStr=Inherit: Inherit via back propagation  SampleTime=-1  PreserveConstantTs=on
  y : Outport  SampleTime=1e-08
  wires:
  u/1 -> Compare/1
  Compare/1 -> y/1
  Constant/1 -> Compare/2

== system gm_UZ_EnDat_be4_segregation/UZ_ENDAT/5timestorage/Triggered Subsystem/Counter Limited ==
  Trigger_emulated : Inport  OutDataTypeStr=boolean  SampleTime=1e-08
  Force to be scalar : SignalSpecification  OutDataTypeStr=uint8  Dimensions=1
  Increment Real World : Subsystem  mask(Real World Value Increment){}
      mask help: Simulink:masks:RealWorldValueIncrement_MD
      mask Display: disp('V++')
  Output : Subsystem
      settings: MinAlgLoopOccurrences=on
  Output_out1 : hdlmdlgenlib/Buffer
  Wrap To Zero : Subsystem  mask(Wrap To Zero){Threshold=double(4)}
      mask prompts: Threshold "Simulink:masks:Threshold_MP"
      mask help: Simulink:masks:WrapToZero_MD
  sigspec : SignalSpecification  OutDataTypeStr=uint8  Dimensions=1
  y : Outport  SampleTime=1e-08  InitialOutput=0
  wires:
  Output_out1/1 -> y/1
  Output/1(out0) -> Output_out1/1, Force to be scalar/1
  sigspec/1 -> Output/1(in0)
  Trigger_emulated/1 -> Output/Enable
  Force to be scalar/1 -> Increment Real World/1(u)
  Increment Real World/1(y) -> Wrap To Zero/1(U)
  Wrap To Zero/1(Y) -> sigspec/1

== system gm_UZ_EnDat_be4_segregation/UZ_ENDAT/CLKCNTER_ACT/Positional_Counter/Increment Stored Integer ==
  u : Inport  OutDataTypeStr=fixdt(0,32,0,'DataTypeOverride', 'Off')  SampleTime=1e-08
  FixPt Constant : Constant  DisableCoverage=on  OutDataTypeStr=Inherit: Inherit via back propagation  SampleTime=-1
  FixPt Data Type Duplicate : DataTypeDuplicate  DisableCoverage=on  NumInputPorts=3
  FixPt Gateway In : DataTypeConversion  DisableCoverage=on  ConvertRealWorld=Stored Integer (SI)  SaturateOnIntegerOverflow=off  RndMeth=Floor
  FixPt Sum1 : Sum  OutDataTypeStr=Inherit: Inherit via back propagation  InputSameDT=on  LockScale=on
  sigspec : SignalSpecification  OutDataTypeStr=uint32  Dimensions=1
  y : Outport  SampleTime=1e-08  InitialOutput=0
  wires:
  sigspec/1 -> FixPt Gateway In/1
  FixPt Sum1/1 -> y/1, FixPt Data Type Duplicate/1
  FixPt Gateway In/1 -> FixPt Data Type Duplicate/3, FixPt Sum1/2
  FixPt Constant/1 -> sigspec/1
  u/1 -> FixPt Data Type Duplicate/2, FixPt Sum1/1

== system gm_UZ_EnDat_be4_segregation/UZ_ENDAT/CLKCNTER_RAMPUP/Positional_Counter/Increment Stored Integer ==
  u : Inport  OutDataTypeStr=fixdt(0,32,0,'DataTypeOverride', 'Off')  SampleTime=1e-08
  FixPt Constant : Constant  DisableCoverage=on  OutDataTypeStr=Inherit: Inherit via back propagation  SampleTime=-1
  FixPt Data Type Duplicate : DataTypeDuplicate  DisableCoverage=on  NumInputPorts=3
  FixPt Gateway In : DataTypeConversion  DisableCoverage=on  ConvertRealWorld=Stored Integer (SI)  SaturateOnIntegerOverflow=off  RndMeth=Floor
  FixPt Sum1 : Sum  OutDataTypeStr=Inherit: Inherit via back propagation  InputSameDT=on  LockScale=on
  sigspec : SignalSpecification  OutDataTypeStr=uint32  Dimensions=1
  y : Outport  SampleTime=1e-08  InitialOutput=0
  wires:
  sigspec/1 -> FixPt Gateway In/1
  FixPt Sum1/1 -> y/1, FixPt Data Type Duplicate/1
  FixPt Gateway In/1 -> FixPt Data Type Duplicate/3, FixPt Sum1/2
  FixPt Constant/1 -> sigspec/1
  u/1 -> FixPt Data Type Duplicate/2, FixPt Sum1/1
